simulink model "XOR_4BIT"  (R2018a)
settings: Solver=VariableStepAuto  StartTime=0.0  StopTime=10.0  RelTol=1e-3
settings Model: Creator=midog  LastModifiedBy=midog

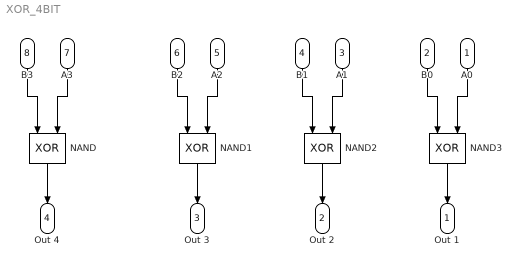
== system XOR_4BIT ==
  A0 : Inport
  B0 : Inport  Port=2
  A1 : Inport  Port=3
  B1 : Inport  Port=4
  A2 : Inport  Port=5
  B2 : Inport  Port=6
  A3 : Inport  Port=7
  B3 : Inport  Port=8
  NAND{,1..3} (4 alike) : Logic  Operator=XOR  IconShape=distinctive  AllPortsSameDT=off  OutDataTypeStr=boolean
  Out 1 : Outport
  Out 2 : Outport  Port=2
  Out 3 : Outport  Port=3
  Out 4 : Outport  Port=4
  wires:
  NAND3/1 -> Out 1/1
  NAND/1 -> Out 4/1
  NAND2/1 -> Out 2/1
  A2/1 -> NAND1/2
  B0/1 -> NAND3/1
  A0/1 -> NAND3/2
  B2/1 -> NAND1/1
  A1/1 -> NAND2/2
  B1/1 -> NAND2/1
  B3/1 -> NAND/1
  NAND1/1 -> Out 3/1
  A3/1 -> NAND/2
